simulink model "wahadlo1"  (R2018a)
settings: Solver=ode1  StartTime=0.0  StopTime=100  FixedStep=0.01  RelTol=1e-3
settings Model: Creator=Koala  LastModifiedBy=Koala

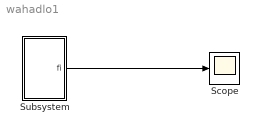
== system wahadlo1 ==
  Scope : Scope
  Subsystem : Subsystem  mask{m=10, l=3, k=1, g=10, fi0=90}
      mask prompts: m "Masa"; l "Długość"; k "Tłumienie"; g "Przyśpieszenie"; fi0 "Kąt początkowy"
  wires:
  Subsystem/1(fi) -> Scope/1

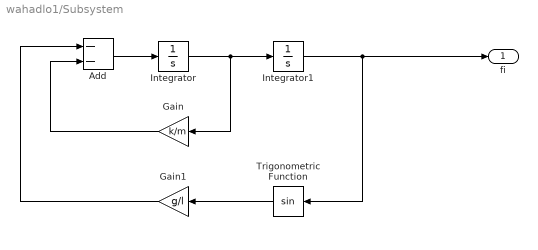
== system wahadlo1/Subsystem ==
  Add : Sum  Inputs=--
  Gain : Gain  Gain=k/m
  Gain1 : Gain  Gain=g/l
  Integrator : Integrator
  Integrator1 : Integrator  InitialCondition=fi0 * pi/180
  Trigonometric Function : Trigonometry
  fi : Outport
  wires:
  Integrator1/1 -> fi/1, Trigonometric Function/1
  Integrator/1 -> Gain/1, Integrator1/1
  Gain1/1 -> Add/1
  Add/1 -> Integrator/1
  Gain/1 -> Add/2
  Trigonometric Function/1 -> Gain1/1
